simulink model "bipedal_robot_CTRL2"  (R2020b)
settings: Solver=ode23  StartTime=0.0  StopTime=Tsim  MaxStep=0.01  RelTol=1e-3  AbsTol=1e-3  EnableMultiTasking=on
values from neighbouring files (symbols this model uses):
  g = 9.80665    [bipedal.m]
  Tfil = Ts*10    (= 0.01)    [bipedal.m]
  total_mass = mlist(1) + ll_mass + rl_mass    [bipedal.m]
  Ts = 1/fs    (= 0.001)    [bipedal.m]
undefined symbols (not defined in the file or in its folder): Base, ctrl_cfg_rem, Fdist, LefAnklePitch, LefAnkleRoll, LefHipPitch, LefHipRoll, LefHipYaw, LefKnee, pg_traj, RigAnklePitch, RigAnkleRoll, RigHipPitch, RigHipRoll, RigHipYaw, RigKnee, sim_floor, Tdist, VAR_DIST, X, Y, Z
libraries: sm_lib x56, biped_lib x39, nesl_utility x18, simulink x3, Contact_Forces_Lib x2, robotmaniplib x1
(part 3 of 4)

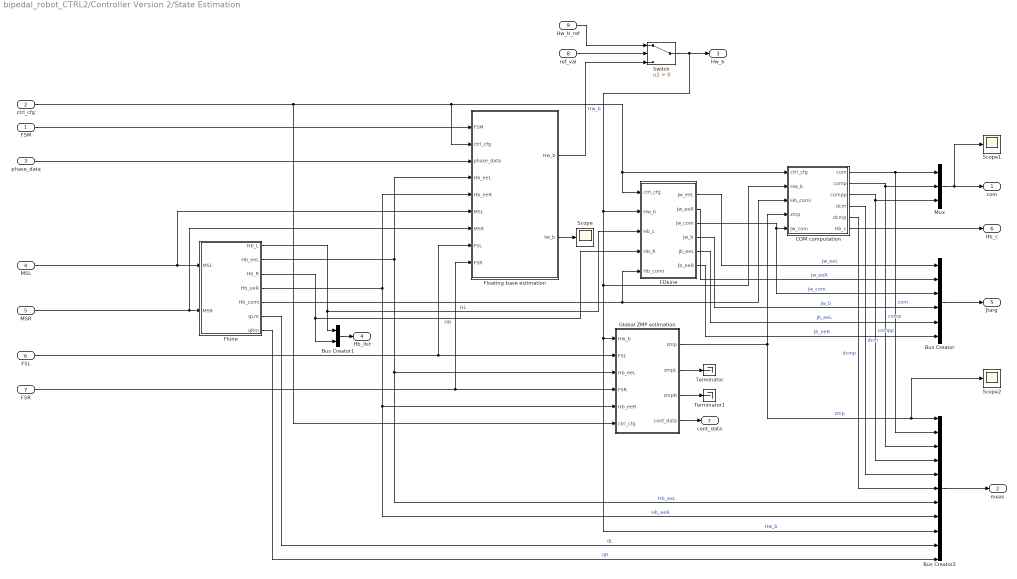
== system bipedal_robot_CTRL2/Controller Version 2/State Estimation ==
  FSM : Inport
  ctrl_cfg : Inport  Port=2
  phase_data : Inport  Port=3  OutDataTypeStr=Bus: ph_data_bus
  MSL : Inport  Port=4
  MSR : Inport  Port=5
  FSL : Inport  Port=6  OutDataTypeStr=Bus: fs_str_bus
  FSR : Inport  Port=7  OutDataTypeStr=Bus: fs_str_bus
  ref_val : Inport  Port=8
  Hw_b_ref : Inport  Port=9
  Bus Creator : BusCreator  Inputs=6  OutDataTypeStr=Bus: jac_bus
  Bus Creator1 : BusCreator  Inputs=2
  Bus Creator2 : BusCreator  Inputs=11  OutDataTypeStr=Bus: meas_bus
  COM computation : MATLAB Function  TreatAsAtomicUnit=on
  FDkine : MATLAB Function  TreatAsAtomicUnit=on
  Fkine : MATLAB Function  TreatAsAtomicUnit=on
  Floating base estimation : MATLAB Function  TreatAsAtomicUnit=on
  Global ZMP estimation : MATLAB Function  TreatAsAtomicUnit=on
  Mux : Mux  Inputs=3
  Scope : Scope
  Scope1 : Scope
  Scope2 : Scope
  Switch : Switch  Criteria=u2 > Threshold
  Terminator : Terminator
  Terminator1 : Terminator
  com : Outport
  meas : Outport  Port=2
  Hw_b : Outport  Port=3
  Hb_list : Outport  Port=4
  Jtarg : Outport  Port=5
  Hb_c : Outport  Port=6
  cont_data : Outport  Port=7
  wires:
  Bus Creator2/1 -> meas/1
  Fkine/7(qRm) -> Bus Creator2/11  "qR"
  Fkine/6(qLm) -> Bus Creator2/10  "qL"
  Fkine/4(Hb_eeR) -> Bus Creator2/8, Global ZMP estimation/5(Hb_eeR), Floating base estimation/5(Hb_eeR)  "Hb_eeR"
  Fkine/2(Hb_eeL) -> Bus Creator2/7, Global ZMP estimation/3(Hb_eeL), Floating base estimation/4(Hb_eeL)  "Hb_eeL"
  COM computation/5(dcmp) -> Bus Creator2/6  "dcmp"
  COM computation/4(dcm) -> Bus Creator2/5  "dcm"
  COM computation/3(compp) -> Bus Creator2/4, Mux/3  "compp"
  COM computation/2(comp) -> Bus Creator2/3, Mux/2  "comp"
  COM computation/1(com) -> Bus Creator2/2, Mux/1  "com"
  Bus Creator1/1 -> Hb_list/1
  Global ZMP estimation/3(zmpR) -> Terminator1/1
  Global ZMP estimation/2(zmpL) -> Terminator/1
  MSR/1 -> Fkine/2(MSR), Floating base estimation/7(MSR)
  MSL/1 -> Fkine/1(MSL), Floating base estimation/6(MSL)
  Global ZMP estimation/1(zmp) -> COM computation/4(zmp), Scope2/1, Bus Creator2/1  "zmp"
  ctrl_cfg/1 -> Global ZMP estimation/6(ctrl_cfg), Floating base estimation/2(ctrl_cfg), COM computation/1(ctrl_cfg), FDkine/1(ctrl_cfg)
  Bus Creator/1 -> Jtarg/1
  FDkine/4(Jw_b) -> Bus Creator/4  "Jw_b"
  FDkine/2(Jw_eeR) -> Bus Creator/2  "Jw_eeR"
  FDkine/1(Jw_eeL) -> Bus Creator/1  "Jw_eeL"
  FDkine/3(Jw_com) -> Bus Creator/3, COM computation/5(Jw_com)  "Jw_com"
  Fkine/5(Hb_comi) -> COM computation/3(Hb_comi), FDkine/5(Hb_comi)
  Switch/1 -> Hw_b/1, FDkine/2(Hw_b), Bus Creator2/9, Global ZMP estimation/1(Hw_b), COM computation/2(Hw_b)  "Hw_b"
  FSM/1 -> Floating base estimation/1(FSM)
  phase_data/1 -> Floating base estimation/3(phase_data)
  Fkine/3(Hb_R) -> FDkine/4(Hb_R), Bus Creator1/2  "HR"
  Fkine/1(Hb_L) -> FDkine/3(Hb_L), Bus Creator1/1  "HL"
  FSR/1 -> Floating base estimation/9(FSR), Global ZMP estimation/4(FSR)
  FSL/1 -> Floating base estimation/8(FSL), Global ZMP estimation/2(FSL)
  Floating base estimation/2(tw_b) -> Scope/1
  ref_val/1 -> Switch/2
  Hw_b_ref/1 -> Switch/1
  Floating base estimation/1(Hw_b) -> Switch/3  "Hw_b"
  FDkine/5(Jb_eeL) -> Bus Creator/5  "Jb_eeL"
  FDkine/6(Jb_eeR) -> Bus Creator/6  "Jb_eeR"
  COM computation/6(Hb_c) -> Hb_c/1
  Mux/1 -> Scope1/1, com/1
  Global ZMP estimation/4(cont_data) -> cont_data/1

== system bipedal_robot_CTRL2/Controller Version 2/Static spring force compensation (internal forces) ==
  ctrl_cfg : Inport
  qL : Inport  Port=2
  qR : Inport  Port=3
  HL_list : Inport  Port=4
  HR_list : Inport  Port=5
  Bungee cord compensation : MATLAB Function  TreatAsAtomicUnit=on
  Gas spring compensation : MATLAB Function  TreatAsAtomicUnit=on
  Sum2 : Sum  Inputs=|++
  Sum3 : Sum  Inputs=|++
  TL : Outport
  TR : Outport  Port=2
  wires:
  qR/1 -> Gas spring compensation/3(MSR)
  qL/1 -> Gas spring compensation/2(MSL)
  HR_list/1 -> Gas spring compensation/5(HR_list), Bungee cord compensation/3(HR_list)
  Gas spring compensation/2(TR) -> Sum3/1
  Gas spring compensation/1(TL) -> Sum2/1
  HL_list/1 -> Gas spring compensation/4(HL_list), Bungee cord compensation/2(HL_list)
  ctrl_cfg/1 -> Gas spring compensation/1(ctrl_cfg), Bungee cord compensation/1(ctrl_cfg)
  Bungee cord compensation/2(TR) -> Sum3/2
  Sum3/1 -> TR/1
  Sum2/1 -> TL/1
  Bungee cord compensation/1(TL) -> Sum2/2

== system bipedal_robot_CTRL2/Controller Version 2/Trajectory Generation ==
  note: 1) Add Subsystem or Model blocks as valid variant choices.
      | 2) You cannot connect blocks at this level. At simulation, connectivity is automatically
      | determined, based on the active variant and port name matching.
  FSM : Inport
  zmp_curr : Inport  Port=2
  com_m : Inport  Port=3
  (C++ impl) : Subsystem  VariantControl=VAR_TG == 2
  Preview Controller (simulink impl) : Subsystem  VariantControl=VAR_TG == 1
  tg_data : Outport  OutDataTypeStr=Bus: tg_out_bus

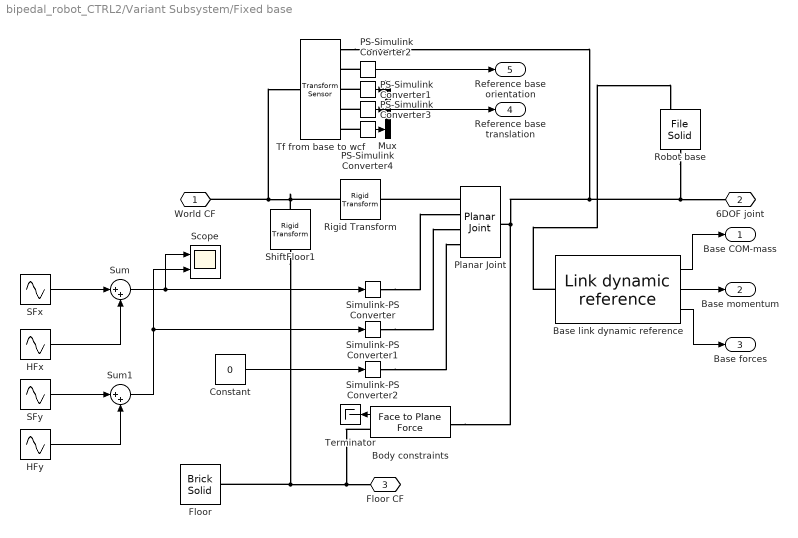
== system bipedal_robot_CTRL2/Variant Subsystem/Fixed base ==
  Base link dynamic reference : biped_lib/Link dynamic reference  M=Base.body.mass  I=Base.body.inertia
  Body constraints : Contact_Forces_Lib/3D/Composite Forces/Face to Plane Force  PlaB_x=sim_floor.dims(1)  PlaB_y=sim_floor.dims(2)  PlaB_z=sim_floor.dims(3)/2  FacF_x=Base.dims(1)  FacF_y=Base.dims(2)  FacF_z=Base.dims(3)/2  FacF_rSph=0.01  force_law_pla2pla=Linear  k_contact_pla2pla=Kcont  b_contact_pla2pla=Dcont  pen_full_damp_F_pla2pla=1e-4  pen_exponent_pla2pla=1  friction_law_pla2pla=Stick-Slip Continuous  mu_kinetic_pla2pla=0.5  mu_static_pla2pla=0.7  v_thr_pla2pla=0.001  vis_on_pla2pla=off  vis_opc_en_box2box=0  vis_len_plaLz=0.005  vis_clr=[0.9 0.2 0.2]  vis_opc=0.7
      settings: SourceProductName=Simscape Multibody Contact Forces Library
  Constant : Constant  Value=0
  Floor : sm_lib/Body Elements/Brick Solid  GraphicAmbientColor=[0.15 0.15 0.15 1.0]  BasedOnType=Density  BrickDimensions=sim_floor.dims  BrickDimensionUnits=m  CenterOfMass=[0 0 0]  CenterOfMassUnits=m  GraphicDiffuseColor=[0.8 0.8 0.8]  Density=1000  DensityUnits=kg/m^3  DoExposeReferenceFrame=on  GraphicEmissiveColor=[0.0 0.0 0.0 1.0]  ExportEntireGeometry=off  SerializedFrames=<Frames/>  MarkerShape=Sphere  MarkerSize=10  GraphicType=FromGeometry  InertiaType=CalculateFromGeometry  Mass=1  MassUnits=kg  MomentsOfInertia=[1 1 1]  MomentsOfInertiaUnits=kg*m^2  GraphicOpacity=1.0  ProductsOfInertia=[0 0 0]  ProductsOfInertiaUnits=kg*m^2  GraphicShininess=75  GraphicSpecularColor=[0.5 0.5 0.5 1.0]  GraphicVisPropType=SimpleVisualProperties
      settings: SourceProductName=Multibody
  HFx : Sin  Amplitude=0.001  Frequency=10  SampleTime=Ts
  HFy : Sin  Amplitude=0.001  Frequency=12  SampleTime=Ts
  Mux : Mux  Inputs=3
  PS-Simulink Converter{1..4} (4 alike) : nesl_utility/PS-Simulink Converter  PhysicalDomain=network_engine_domain  SubClassName=ps_output  LeftPortType=input  RightPortType=output  PseudoPeriodic=off  Frequencies=[]  Unit=1  AffineConversion=off
  Planar Joint : sm_lib/Joints/Planar Joint  JointMode=Normal  SenseConstraintForce=off  SenseConstraintForceX=off  SenseConstraintForceY=off  SenseConstraintForceZ=off  SenseConstraintTorque=off  SenseConstraintTorqueX=off  SenseConstraintTorqueY=off  SenseConstraintTorqueZ=off  SenseTotalForce=off  SenseTotalForceX=off  SenseTotalForceY=off  SenseTotalForceZ=off  SenseTotalTorque=off  SenseTotalTorqueX=off  SenseTotalTorqueY=off  SenseTotalTorqueZ=off  CompositeWrenchDir=FollowerOnBase  CompositeWrenchFrame=BaseFrame  PxEquilibriumPosition=0  PxEquilibriumPositionUnits=m  PxSpringStiffness=1000  PxSpringStiffnessUnits=N/m  PxDampingCoefficient=100  PxDampingCoefficientUnits=N/(m/s)  PxTorqueActuationMode=ComputedTorque  PxMotionActuationMode=InputMotion  PxSensePosition=off  PxSenseVelocity=off  PxSenseAcceleration=off  PxSenseTorqueForce=off  PxSenseLowerLimitTorqueForce=off  PxSenseUpperLimitTorqueForce=off  PxLowerLimitSpecify=off  PxLowerLimitBound=-1  PxLowerLimitBoundUnits=m  PxLowerLimitStiffness=1e6  PxLowerLimitStiffnessUnits=N/m  PxLowerLimitDamping=1e3  PxLowerLimitDampingUnits=N/(m/s)  PxLowerLimitTransitionRegionWidth=1e-4  PxLowerLimitTransitionRegionWidthUnits=m  PxUpperLimitSpecify=off  PxUpperLimitBound=1  PxUpperLimitBoundUnits=m  PxUpperLimitStiffness=1e6  PxUpperLimitStiffnessUnits=N/m  PxUpperLimitDamping=1e3  PxUpperLimitDampingUnits=N/(m/s)  PxUpperLimitTransitionRegionWidth=1e-4  PxUpperLimitTransitionRegionWidthUnits=m  PxPositionTargetSpecify=off  PxPositionTargetPriority=High  PxPositionTargetValue=0  PxPositionTargetValueUnits=m  PxVelocityTargetSpecify=off  PxVelocityTargetPriority=High  PxVelocityTargetValue=0  PxVelocityTargetValueUnits=m/s  PyEquilibriumPosition=0  PyEquilibriumPositionUnits=m  PySpringStiffness=1000  PySpringStiffnessUnits=N/m  PyDampingCoefficient=100  PyDampingCoefficientUnits=N/(m/s)  PyTorqueActuationMode=ComputedTorque  PyMotionActuationMode=InputMotion  PySensePosition=off  PySenseVelocity=off  PySenseAcceleration=off  PySenseTorqueForce=off  PySenseLowerLimitTorqueForce=off  PySenseUpperLimitTorqueForce=off  PyLowerLimitSpecify=off  PyLowerLimitBound=-1  PyLowerLimitBoundUnits=m  PyLowerLimitStiffness=1e6  PyLowerLimitStiffnessUnits=N/m  PyLowerLimitDamping=1e3  PyLowerLimitDampingUnits=N/(m/s)  PyLowerLimitTransitionRegionWidth=1e-4  PyLowerLimitTransitionRegionWidthUnits=m  PyUpperLimitSpecify=off  PyUpperLimitBound=1  PyUpperLimitBoundUnits=m  PyUpperLimitStiffness=1e6  PyUpperLimitStiffnessUnits=N/m  PyUpperLimitDamping=1e3  PyUpperLimitDampingUnits=N/(m/s)  PyUpperLimitTransitionRegionWidth=1e-4  PyUpperLimitTransitionRegionWidthUnits=m  PyPositionTargetSpecify=off  PyPositionTargetPriority=High  PyPositionTargetValue=0  PyPositionTargetValueUnits=m  PyVelocityTargetSpecify=off  PyVelocityTargetPriority=High  PyVelocityTargetValue=0  PyVelocityTargetValueUnits=m/s  RzEquilibriumPosition=0  RzEquilibriumPositionUnits=deg  RzSpringStiffness=1000  RzSpringStiffnessUnits=N*m/deg  RzDampingCoefficient=100  RzDampingCoefficientUnits=N*m/(deg/s)  RzTorqueActuationMode=ComputedTorque  RzMotionActuationMode=InputMotion  RzSensePosition=off  RzSenseVelocity=off  RzSenseAcceleration=off  RzSenseTorqueForce=off  RzSenseLowerLimitTorqueForce=off  RzSenseUpperLimitTorqueForce=off  RzLowerLimitSpecify=off  RzLowerLimitBound=-90  RzLowerLimitBoundUnits=deg  RzLowerLimitStiffness=1e4  RzLowerLimitStiffnessUnits=N*m/deg  RzLowerLimitDamping=10  RzLowerLimitDampingUnits=N*m/(deg/s)  RzLowerLimitTransitionRegionWidth=0.1  RzLowerLimitTransitionRegionWidthUnits=deg  RzUpperLimitSpecify=off  RzUpperLimitBound=90  RzUpperLimitBoundUnits=deg  RzUpperLimitStiffness=1e4  RzUpperLimitStiffnessUnits=N*m/deg  RzUpperLimitDamping=10  RzUpperLimitDampingUnits=N*m/(deg/s)  RzUpperLimitTransitionRegionWidth=0.1  RzUpperLimitTransitionRegionWidthUnits=deg  RzPositionTargetSpecify=off  RzPositionTargetPriority=High  RzPositionTargetValue=0  RzPositionTargetValueUnits=deg  RzVelocityTargetSpecify=off  RzVelocityTargetPriority=High  RzVelocityTargetValue=0  RzVelocityTargetValueUnits=deg/s
  Rigid Transform : sm_lib/Frames and Transforms/Rigid Transform  TranslationMethod=Cartesian  TranslationStandardOffset=Base.Xinit  TranslationLengthUnit=m  TranslationStandardAxis=+Z  TranslationCartesianOffset=Base.Xinit  TranslationROffset=0  TranslationROffsetUnits=m  TranslationZOffset=0  TranslationZOffsetUnits=m  TranslationThetaOffset=0  TranslationThetaOffsetUnits=deg  RotationMethod=None  RotationAngleUnits=deg  RotationStandardAxis=+Z  RotationAngle=0.0  RotationArbitraryAxis=[0 0 1]  FollAlignAxisA=+X  BaseAlignAxisA=+Y  FollAlignAxisB=+Y  BaseAlignAxisB=+Z  RotationSequenceAxes=FollowerAxes  RotationSequence=XYX  RotationSequenceAngles=[0 0 0]  RotationSequenceAnglesUnits=deg  RotationMatrix=[1 0 0; 0 1 0; 0 0 1]
  Robot base : sm_lib/Body Elements/File Solid  ExtGeomFileName=Base.stl  UnitType=Custom  ExtGeomFileUnits=mm  StepReaderType=HEX  ExportConvexHullGeometry=on  InertiaType=Custom  Mass=Base.body.mass  MassUnits=kg  CenterOfMass=Base.body.com  CenterOfMassUnits=m  MomentsOfInertia=Base.body.inertia(1:3)  MomentsOfInertiaUnits=kg*m^2  ProductsOfInertia=Base.body.inertia(4:6)  ProductsOfInertiaUnits=kg*m^2  BasedOnType=Mass  Density=1000  DensityUnits=kg/m^3  DoExposeReferenceFrame=on  SerializedFrames=<Frames><Frame><Id>Frame1</Id><Value><Name>COM</Name><Origin><Source>CenterOfMassFrame</Source><FeatureName></FeatureName></Origin><PrimaryAxis><DefinedDirection>+Z</DefinedDirection><Source>ReferenceFrame</Source><SourceDirection>+Z</SourceDirection><FeatureName></FeatureName></PrimaryAxis><SecondaryAxis><DefinedDirection>+X</DefinedDirection><Source>ReferenceFrame</Source><SourceDirection>+X</SourceDirection><FeatureName></FeatureName></SecondaryAxis></Value></Frame></Frames>  GraphicType=FromGeometry  MarkerShape=Sphere  MarkerSize=10  GraphicVisPropType=SimpleVisualProperties  GraphicDiffuseColor=[0.5 0.5 0.5]  GraphicSpecularColor=[0.5 0.5 0.5 1.0]  GraphicAmbientColor=[0.15 0.15 0.15 1.0]  GraphicEmissiveColor=[0.0 0.0 0.0 1.0]  GraphicShininess=75  GraphicOpacity=1.0
  SFx : Sin  Amplitude=0.2  Frequency=0.5  SampleTime=Ts
  SFy : Sin  Amplitude=0.1  SampleTime=Ts
  Scope : Scope  NumInputPorts=2
  ShiftFloor1 : sm_lib/Frames and Transforms/Rigid Transform  TranslationMethod=StandardAxis  TranslationStandardOffset=-sim_floor.dims(3)/2*5  TranslationLengthUnit=m  TranslationStandardAxis=+Z  TranslationCartesianOffset=[0 0 0]  TranslationROffset=0  TranslationROffsetUnits=m  TranslationZOffset=0  TranslationZOffsetUnits=m  TranslationThetaOffset=0  TranslationThetaOffsetUnits=deg  RotationMethod=None  RotationAngleUnits=deg  RotationStandardAxis=+Z  RotationAngle=0.0  RotationArbitraryAxis=[0 0 1]  FollAlignAxisA=+X  BaseAlignAxisA=+Y  FollAlignAxisB=+Y  BaseAlignAxisB=+Z  RotationSequenceAxes=FollowerAxes  RotationSequence=XYX  RotationSequenceAngles=[0 0 0]  RotationSequenceAnglesUnits=deg  RotationMatrix=[1 0 0; 0 1 0; 0 0 1]
  Simulink-PS Converter : nesl_utility/Simulink-PS Converter  PhysicalDomain=network_engine_domain  SubClassName=ps_input  LeftPortType=input  RightPortType=output  PseudoPeriodic=off  Frequencies=[]  NoiseDistribution=none  NoiseParameters=[]  Unit=1  AffineConversion=off  FilteringAndDerivatives=filter  SimscapeFilterOrder=2  InputFilterTimeConstant=0.001  UdotUserProvided=0
      settings: SourceProductName=Utilities
  Simulink-PS Converter1 : nesl_utility/Simulink-PS Converter  PhysicalDomain=network_engine_domain  SubClassName=ps_input  LeftPortType=input  RightPortType=output  PseudoPeriodic=off  Frequencies=[]  NoiseDistribution=none  NoiseParameters=[]  Unit=1  AffineConversion=off  FilteringAndDerivatives=filter  SimscapeFilterOrder=2  InputFilterTimeConstant=0.001  UdotUserProvided=0
      settings: SourceProductName=Utilities
  Simulink-PS Converter2 : nesl_utility/Simulink-PS Converter  PhysicalDomain=network_engine_domain  SubClassName=ps_input  LeftPortType=input  RightPortType=output  PseudoPeriodic=off  Frequencies=[]  NoiseDistribution=none  NoiseParameters=[]  Unit=1  AffineConversion=off  FilteringAndDerivatives=filter  SimscapeFilterOrder=2  InputFilterTimeConstant=0.001  UdotUserProvided=0
      settings: SourceProductName=Utilities
  Sum : Sum  Inputs=|++
  Sum1 : Sum  Inputs=|++
  Terminator : Terminator
  Tf from base to wcf : sm_lib/Frames and Transforms/Transform Sensor  MeasurementFrame=World  SenseAngle=off  SenseAxis=off  SenseAngle1=off  SenseAngle2=off  SenseAngle3=off  SenseQ=off  SenseR=on  SenseOmegaX=off  SenseOmegaY=off  SenseOmegaZ=off  SenseOmega1=off  SenseOmega2=off  SenseOmega3=off  SenseQDot=off  SenseRDot=off  SenseAlphaX=off  SenseAlphaY=off  SenseAlphaZ=off  SenseAlpha1=off  SenseAlpha2=off  SenseAlpha3=off  SenseQDDot=off  SenseRDDot=off  SenseX=on  SenseY=on  SenseZ=on  SenseRad=off  SenseAzim=off  SenseDist=off  SenseInc=off  SenseXDot=off  SenseYDot=off  SenseZDot=off  SenseRadDot=off  SenseAzimDot=off  SenseDistDot=off  SenseIncDot=off  SenseXDDot=off  SenseYDDot=off  SenseZDDot=off  SenseRadDDot=off  SenseAzimDDot=off  SenseDistDDot=off  SenseIncDDot=off
  World CF : PMIOPort  Side=Left
  6DOF joint : PMIOPort  Port=2  Side=Right
  Floor CF : PMIOPort  Port=3  Side=Right
  Base COM-mass : Outport
  Base momentum : Outport  Port=2
  Base forces : Outport  Port=3
  Reference base translation : Outport  Port=4
  Reference base orientation : Outport  Port=5
  wires:
  Mux/1 -> Reference base translation/1
  PS-Simulink Converter4/1 -> Mux/3
  PS-Simulink Converter1/1 -> Mux/1
  PS-Simulink Converter3/1 -> Mux/2
  PS-Simulink Converter2/1 -> Reference base orientation/1
  Base link dynamic reference/3 -> Base forces/1
  Base link dynamic reference/2 -> Base momentum/1
  Base link dynamic reference/1 -> Base COM-mass/1
  Body constraints/1 -> Terminator/1
  Sum/1 -> Simulink-PS Converter/1, Scope/1
  Sum1/1 -> Simulink-PS Converter1/1, Scope/2
  Constant/1 -> Simulink-PS Converter2/1
  SFy/1 -> Sum1/1
  HFy/1 -> Sum1/2
  HFx/1 -> Sum/2
  SFx/1 -> Sum/1
  connections:
  Base link dynamic reference/LConn1 -- Robot base/LConn1
  PS-Simulink Converter4/LConn1 -- Tf from base to wcf/RConn5
  PS-Simulink Converter3/LConn1 -- Tf from base to wcf/RConn4
  PS-Simulink Converter1/LConn1 -- Tf from base to wcf/RConn3
  PS-Simulink Converter2/LConn1 -- Tf from base to wcf/RConn2
  Body constraints/RConn1 -- Floor CF/RConn1 -- Floor/RConn1 -- ShiftFloor1/RConn1
  Robot base/RConn1 -- 6DOF joint/RConn1 -- Tf from base to wcf/RConn1 -- Body constraints/LConn1 -- Planar Joint/RConn1
  ShiftFloor1/LConn1 -- World CF/RConn1 -- Tf from base to wcf/LConn1 -- Rigid Transform/LConn1
  Planar Joint/LConn1 -- Rigid Transform/RConn1
  Simulink-PS Converter/RConn1 -- Planar Joint/LConn2
  Simulink-PS Converter1/RConn1 -- Planar Joint/LConn3
  Simulink-PS Converter2/RConn1 -- Planar Joint/LConn4

== system bipedal_robot_CTRL2/Variant Subsystem/Floating base ==
  6-DOF Joint : sm_lib/Joints/6-DOF Joint  JointMode=Normal  SenseConstraintForce=off  SenseConstraintForceX=off  SenseConstraintForceY=off  SenseConstraintForceZ=off  SenseConstraintTorque=off  SenseConstraintTorqueX=off  SenseConstraintTorqueY=off  SenseConstraintTorqueZ=off  SenseTotalForce=off  SenseTotalForceX=off  SenseTotalForceY=off  SenseTotalForceZ=off  SenseTotalTorque=off  SenseTotalTorqueX=off  SenseTotalTorqueY=off  SenseTotalTorqueZ=off  CompositeWrenchDir=FollowerOnBase  CompositeWrenchFrame=BaseFrame  PxEquilibriumPosition=0  PxEquilibriumPositionUnits=m  PxSpringStiffness=0  PxSpringStiffnessUnits=N/m  PxDampingCoefficient=0  PxDampingCoefficientUnits=N/(m/s)  PxTorqueActuationMode=NoTorque  PxMotionActuationMode=ComputedMotion  PxSensePosition=off  PxSenseVelocity=off  PxSenseAcceleration=off  PxSenseTorqueForce=off  PxSenseLowerLimitTorqueForce=off  PxSenseUpperLimitTorqueForce=off  PxLowerLimitSpecify=off  PxLowerLimitBound=-1  PxLowerLimitBoundUnits=m  PxLowerLimitStiffness=1e6  PxLowerLimitStiffnessUnits=N/m  PxLowerLimitDamping=1e3  PxLowerLimitDampingUnits=N/(m/s)  PxLowerLimitTransitionRegionWidth=1e-4  PxLowerLimitTransitionRegionWidthUnits=m  PxUpperLimitSpecify=off  PxUpperLimitBound=1  PxUpperLimitBoundUnits=m  PxUpperLimitStiffness=1e6  PxUpperLimitStiffnessUnits=N/m  PxUpperLimitDamping=1e3  PxUpperLimitDampingUnits=N/(m/s)  PxUpperLimitTransitionRegionWidth=1e-4  PxUpperLimitTransitionRegionWidthUnits=m  PxPositionTargetSpecify=on  PxPositionTargetPriority=High  PxPositionTargetValue=Base.Xinit(1)  PxPositionTargetValueUnits=m  PxVelocityTargetSpecify=off  PxVelocityTargetPriority=High  PxVelocityTargetValue=0  PxVelocityTargetValueUnits=m/s  PyEquilibriumPosition=0  PyEquilibriumPositionUnits=m  PySpringStiffness=0  PySpringStiffnessUnits=N/m  PyDampingCoefficient=0  PyDampingCoefficientUnits=N/(m/s)  PyTorqueActuationMode=NoTorque  PyMotionActuationMode=ComputedMotion  PySensePosition=off  PySenseVelocity=off  PySenseAcceleration=off  PySenseTorqueForce=off  PySenseLowerLimitTorqueForce=off  PySenseUpperLimitTorqueForce=off  PyLowerLimitSpecify=off  PyLowerLimitBound=-1  PyLowerLimitBoundUnits=m  PyLowerLimitStiffness=1e6  PyLowerLimitStiffnessUnits=N/m  PyLowerLimitDamping=1e3  PyLowerLimitDampingUnits=N/(m/s)  PyLowerLimitTransitionRegionWidth=1e-4  PyLowerLimitTransitionRegionWidthUnits=m  PyUpperLimitSpecify=off  PyUpperLimitBound=1  PyUpperLimitBoundUnits=m  PyUpperLimitStiffness=1e6  PyUpperLimitStiffnessUnits=N/m  PyUpperLimitDamping=1e3  PyUpperLimitDampingUnits=N/(m/s)  PyUpperLimitTransitionRegionWidth=1e-4  PyUpperLimitTransitionRegionWidthUnits=m  PyPositionTargetSpecify=on  PyPositionTargetPriority=High  PyPositionTargetValue=Base.Xinit(2)  PyPositionTargetValueUnits=m  PyVelocityTargetSpecify=off  PyVelocityTargetPriority=High  PyVelocityTargetValue=0  PyVelocityTargetValueUnits=m/s  PzEquilibriumPosition=0  PzEquilibriumPositionUnits=m  PzSpringStiffness=0  PzSpringStiffnessUnits=N/m  PzDampingCoefficient=0  PzDampingCoefficientUnits=N/(m/s)  PzTorqueActuationMode=NoTorque  PzMotionActuationMode=ComputedMotion  PzSensePosition=off  PzSenseVelocity=off  PzSenseAcceleration=off  PzSenseTorqueForce=off  PzSenseLowerLimitTorqueForce=off  PzSenseUpperLimitTorqueForce=off  PzLowerLimitSpecify=off  PzLowerLimitBound=0  PzLowerLimitBoundUnits=m  PzLowerLimitStiffness=1e6  PzLowerLimitStiffnessUnits=N/m  PzLowerLimitDamping=1e3  PzLowerLimitDampingUnits=N/(m/s)  PzLowerLimitTransitionRegionWidth=1e-4  PzLowerLimitTransitionRegionWidthUnits=m  PzUpperLimitSpecify=off  PzUpperLimitBound=1  PzUpperLimitBoundUnits=m  PzUpperLimitStiffness=1e6  PzUpperLimitStiffnessUnits=N/m  PzUpperLimitDamping=1e3  PzUpperLimitDampingUnits=N/(m/s)  PzUpperLimitTransitionRegionWidth=1e-4  PzUpperLimitTransitionRegionWidthUnits=m  PzPositionTargetSpecify=on  PzPositionTargetPriority=High  PzPositionTargetValue=Base.Xinit(3)  PzPositionTargetValueUnits=m  PzVelocityTargetSpecify=off  PzVelocityTargetPriority=High  PzVelocityTargetValue=0  PzVelocityTargetValueUnits=m/s  SphDefPosRotationMethod=None  SphDefPosRotationAngleUnits=deg  SphDefPosRotationStandardAxis=+Z  SphDefPosRotationAngle=0.0  SphDefPosRotationArbitraryAxis=[0 0 1]  SphDefPosFollAlignAxisA=+X  SphDefPosBaseAlignAxisA=+Y  SphDefPosFollAlignAxisB=+Y  SphDefPosBaseAlignAxisB=+Z  SphDefPosRotationSequenceAxes=FollowerAxes  SphDefPosRotationSequence=XYX  SphDefPosRotationSequenceAngles=[0 0 0]  SphDefPosRotationSequenceAnglesUnits=deg  SphDefPosRotationMatrix=[1 0 0; 0 1 0; 0 0 1]  SphEqPosRotationMethod=None  SphEqPosRotationAngleUnits=deg  SphEqPosRotationStandardAxis=+Z  SphEqPosRotationAngle=0.0  SphEqPosRotationArbitraryAxis=[0 0 1]  SphEqPosFollAlignAxisA=+X  SphEqPosBaseAlignAxisA=+Y  SphEqPosFollAlignAxisB=+Y  SphEqPosBaseAlignAxisB=+Z  SphEqPosRotationSequenceAxes=FollowerAxes  SphEqPosRotationSequence=XYX  SphEqPosRotationSequenceAngles=[0 0 0]  SphEqPosRotationSequenceAnglesUnits=deg  SphEqPosRotationMatrix=[1 0 0; 0 1 0; 0 0 1]  SphSpringStiffness=0  SphSpringStiffnessUnits=N*m/deg  SphDampingCoefficient=0  SphDampingCoefficientUnits=N*m/(deg/s)  SphActuateTorqueX=off  SphActuateTorqueY=off  SphActuateTorqueZ=off  SphActuateTorque=off  SphTorqueActuationMode=NoTorque  SphMotionActuationMode=ComputedMotion  SphActuationFrame=BaseFrame  SphSensePosition=off  SphSenseVelocityX=off  SphSenseVelocityY=off  SphSenseVelocityZ=off  SphSenseVelocity=off  SphSenseAccelerationX=off  SphSenseAccelerationY=off  SphSenseAccelerationZ=off  SphSenseAcceleration=off  SphSenseTorqueX=off  SphSenseTorqueY=off  SphSenseTorqueZ=off  SphSenseTorqueForce=off  SphSenseLowerLimitTorqueMag=off  SphSenseUpperLimitTorqueMag=off  SphSensingFrame=BaseFrame  SphLowerLimitSpecify=off  SphLowerLimitBound=15  SphLowerLimitBoundUnits=deg  SphLowerLimitStiffness=1e4  SphLowerLimitStiffnessUnits=N*m/deg  SphLowerLimitDamping=10  SphLowerLimitDampingUnits=N*m/(deg/s)  SphLowerLimitTransitionRegionWidth=0.1  SphLowerLimitTransitionRegionWidthUnits=deg  SphUpperLimitSpecify=off  SphUpperLimitBound=45  SphUpperLimitBoundUnits=deg  SphUpperLimitStiffness=1e4  SphUpperLimitStiffnessUnits=N*m/deg  SphUpperLimitDamping=10  SphUpperLimitDampingUnits=N*m/(deg/s)  SphUpperLimitTransitionRegionWidth=0.1  SphUpperLimitTransitionRegionWidthUnits=deg  SphPositionTargetRotationMethod=StandardAxis  SphPositionTargetRotationAngleUnits=rad  SphPositionTargetRotationStandardAxis=+Y  SphPositionTargetRotationAngle=0  SphPositionTargetRotationArbitraryAxis=[0 0 1]  SphPositionTargetFollAlignAxisA=+X  SphPositionTargetBaseAlignAxisA=+Y  SphPositionTargetFollAlignAxisB=+Y  SphPositionTargetBaseAlignAxisB=+Z  SphPositionTargetRotationSequenceAxes=FollowerAxes  SphPositionTargetRotationSequence=XYX  SphPositionTargetRotationSequenceAngles=[0 0 0]  SphPositionTargetRotationSequenceAnglesUnits=deg  SphPositionTargetRotationMatrix=[1 0 0; 0 1 0; 0 0 1]  SphPositionTargetSpecify=on  SphPositionTargetPriority=High  SphVelocityTargetValue=[0 0 0]  SphVelocityTargetValueUnits=deg/s  SphVelocityTargetSpecify=off  SphVelocityTargetPriority=High  SphVelocityTargetInFollowerFrame=on
  Base link dynamic reference : biped_lib/Link dynamic reference  M=Base.body.mass  I=Base.body.inertia
  Body constraints : Contact_Forces_Lib/3D/Composite Forces/Face to Plane Force  PlaB_x=sim_floor.dims(1)  PlaB_y=sim_floor.dims(2)  PlaB_z=sim_floor.dims(3)/2  FacF_x=Base.dims(1)  FacF_y=Base.dims(2)  FacF_z=Base.dims(3)/2  FacF_rSph=0.01  force_law_pla2pla=Linear  k_contact_pla2pla=Kcont  b_contact_pla2pla=Dcont  pen_full_damp_F_pla2pla=1e-4  pen_exponent_pla2pla=1  friction_law_pla2pla=Stick-Slip Continuous  mu_kinetic_pla2pla=0.5  mu_static_pla2pla=0.7  v_thr_pla2pla=0.001  vis_on_pla2pla=off  vis_opc_en_box2box=0  vis_len_plaLz=0.005  vis_clr=[0.9 0.2 0.2]  vis_opc=0.7
      settings: SourceProductName=Simscape Multibody Contact Forces Library
  Disturbance generator : Subsystem
  Floor : sm_lib/Body Elements/Brick Solid  GraphicAmbientColor=[0.15 0.15 0.15 1.0]  BasedOnType=Density  BrickDimensions=sim_floor.dims  BrickDimensionUnits=m  CenterOfMass=[0 0 0]  CenterOfMassUnits=m  GraphicDiffuseColor=[0.8 0.8 0.8]  Density=1000  DensityUnits=kg/m^3  DoExposeReferenceFrame=on  GraphicEmissiveColor=[0.0 0.0 0.0 1.0]  ExportEntireGeometry=off  SerializedFrames=<Frames/>  MarkerShape=Sphere  MarkerSize=10  GraphicType=FromGeometry  InertiaType=CalculateFromGeometry  Mass=1  MassUnits=kg  MomentsOfInertia=[1 1 1]  MomentsOfInertiaUnits=kg*m^2  GraphicOpacity=1.0  ProductsOfInertia=[0 0 0]  ProductsOfInertiaUnits=kg*m^2  GraphicShininess=75  GraphicSpecularColor=[0.5 0.5 0.5 1.0]  GraphicVisPropType=SimpleVisualProperties
      settings: SourceProductName=Multibody
  Mux : Mux  Inputs=3
  PS-Simulink Converter{1..4} (4 alike) : nesl_utility/PS-Simulink Converter  PhysicalDomain=network_engine_domain  SubClassName=ps_output  LeftPortType=input  RightPortType=output  PseudoPeriodic=off  Frequencies=[]  Unit=1  AffineConversion=off
  Rigid Transform : sm_lib/Frames and Transforms/Rigid Transform  TranslationMethod=StandardAxis  TranslationStandardOffset=0  TranslationLengthUnit=m  TranslationStandardAxis=+Z  TranslationCartesianOffset=[0 0 0]  TranslationROffset=0  TranslationROffsetUnits=m  TranslationZOffset=0  TranslationZOffsetUnits=m  TranslationThetaOffset=0  TranslationThetaOffsetUnits=deg  RotationMethod=None  RotationAngleUnits=deg  RotationStandardAxis=+Z  RotationAngle=0.0  RotationArbitraryAxis=[0 0 1]  FollAlignAxisA=+X  BaseAlignAxisA=+Y  FollAlignAxisB=+Y  BaseAlignAxisB=+Z  RotationSequenceAxes=FollowerAxes  RotationSequence=XYX  RotationSequenceAngles=[0 0 0]  RotationSequenceAnglesUnits=deg  RotationMatrix=[1 0 0; 0 1 0; 0 0 1]
  Robot base : sm_lib/Body Elements/File Solid  ExtGeomFileName=Base.stl  UnitType=Custom  ExtGeomFileUnits=mm  StepReaderType=HEX  ExportConvexHullGeometry=on  InertiaType=Custom  Mass=Base.body.mass  MassUnits=kg  CenterOfMass=Base.body.com  CenterOfMassUnits=m  MomentsOfInertia=Base.body.inertia(1:3)  MomentsOfInertiaUnits=kg*m^2  ProductsOfInertia=Base.body.inertia(4:6)  ProductsOfInertiaUnits=kg*m^2  BasedOnType=Mass  Density=1000  DensityUnits=kg/m^3  DoExposeReferenceFrame=on  SerializedFrames=<Frames><Frame><Id>Frame1</Id><Value><Name>COM</Name><Origin><Source>CenterOfMassFrame</Source><FeatureName></FeatureName></Origin><PrimaryAxis><DefinedDirection>+Z</DefinedDirection><Source>ReferenceFrame</Source><SourceDirection>+Z</SourceDirection><FeatureName></FeatureName></PrimaryAxis><SecondaryAxis><DefinedDirection>+X</DefinedDirection><Source>ReferenceFrame</Source><SourceDirection>+X</SourceDirection><FeatureName></FeatureName></SecondaryAxis></Value></Frame></Frames>  GraphicType=FromGeometry  MarkerShape=Sphere  MarkerSize=10  GraphicVisPropType=SimpleVisualProperties  GraphicDiffuseColor=[0.5 0.5 0.5]  GraphicSpecularColor=[0.5 0.5 0.5 1.0]  GraphicAmbientColor=[0.15 0.15 0.15 1.0]  GraphicEmissiveColor=[0.0 0.0 0.0 1.0]  GraphicShininess=75  GraphicOpacity=1.0
  ShiftFloor1 : sm_lib/Frames and Transforms/Rigid Transform  TranslationMethod=StandardAxis  TranslationStandardOffset=-sim_floor.dims(3)/2  TranslationLengthUnit=m  TranslationStandardAxis=+Z  TranslationCartesianOffset=[0 0 0]  TranslationROffset=0  TranslationROffsetUnits=m  TranslationZOffset=0  TranslationZOffsetUnits=m  TranslationThetaOffset=0  TranslationThetaOffsetUnits=deg  RotationMethod=None  RotationAngleUnits=deg  RotationStandardAxis=+Z  RotationAngle=0.0  RotationArbitraryAxis=[0 0 1]  FollAlignAxisA=+X  BaseAlignAxisA=+Y  FollAlignAxisB=+Y  BaseAlignAxisB=+Z  RotationSequenceAxes=FollowerAxes  RotationSequence=XYX  RotationSequenceAngles=[0 0 0]  RotationSequenceAnglesUnits=deg  RotationMatrix=[1 0 0; 0 1 0; 0 0 1]
  Terminator : Terminator
  Tf from base to wcf : sm_lib/Frames and Transforms/Transform Sensor  MeasurementFrame=World  SenseAngle=off  SenseAxis=off  SenseAngle1=off  SenseAngle2=off  SenseAngle3=off  SenseQ=off  SenseR=on  SenseOmegaX=off  SenseOmegaY=off  SenseOmegaZ=off  SenseOmega1=off  SenseOmega2=off  SenseOmega3=off  SenseQDot=off  SenseRDot=off  SenseAlphaX=off  SenseAlphaY=off  SenseAlphaZ=off  SenseAlpha1=off  SenseAlpha2=off  SenseAlpha3=off  SenseQDDot=off  SenseRDDot=off  SenseX=on  SenseY=on  SenseZ=on  SenseRad=off  SenseAzim=off  SenseDist=off  SenseInc=off  SenseXDot=off  SenseYDot=off  SenseZDot=off  SenseRadDot=off  SenseAzimDot=off  SenseDistDot=off  SenseIncDot=off  SenseXDDot=off  SenseYDDot=off  SenseZDDot=off  SenseRadDDot=off  SenseAzimDDot=off  SenseDistDDot=off  SenseIncDDot=off
  World CF : PMIOPort  Side=Left
  6DOF joint : PMIOPort  Port=2  Side=Right
  Floor CF : PMIOPort  Port=3  Side=Right
  Base COM-mass : Outport
  Base momentum : Outport  Port=2
  Base forces : Outport  Port=3
  Reference base translation : Outport  Port=4
  Reference base orientation : Outport  Port=5
  wires:
  Body constraints/1 -> Terminator/1
  Base link dynamic reference/1 -> Base COM-mass/1
  Base link dynamic reference/2 -> Base momentum/1
  Base link dynamic reference/3 -> Base forces/1
  PS-Simulink Converter2/1 -> Reference base orientation/1
  PS-Simulink Converter3/1 -> Mux/2
  PS-Simulink Converter1/1 -> Mux/1
  PS-Simulink Converter4/1 -> Mux/3
  Mux/1 -> Reference base translation/1
  connections:
  Rigid Transform/LConn1 -- Tf from base to wcf/LConn1 -- World CF/RConn1 -- ShiftFloor1/LConn1
  Rigid Transform/RConn1 -- 6-DOF Joint/LConn1
  6-DOF Joint/RConn1 -- Body constraints/LConn1 -- Disturbance generator/RConn1 -- Tf from base to wcf/RConn1 -- Robot base/RConn1 -- 6DOF joint/RConn1
  ShiftFloor1/RConn1 -- Floor/RConn1 -- Floor CF/RConn1 -- Body constraints/RConn1
  PS-Simulink Converter2/LConn1 -- Tf from base to wcf/RConn2
  PS-Simulink Converter1/LConn1 -- Tf from base to wcf/RConn3
  PS-Simulink Converter3/LConn1 -- Tf from base to wcf/RConn4
  PS-Simulink Converter4/LConn1 -- Tf from base to wcf/RConn5
  Base link dynamic reference/LConn1 -- Robot base/LConn1

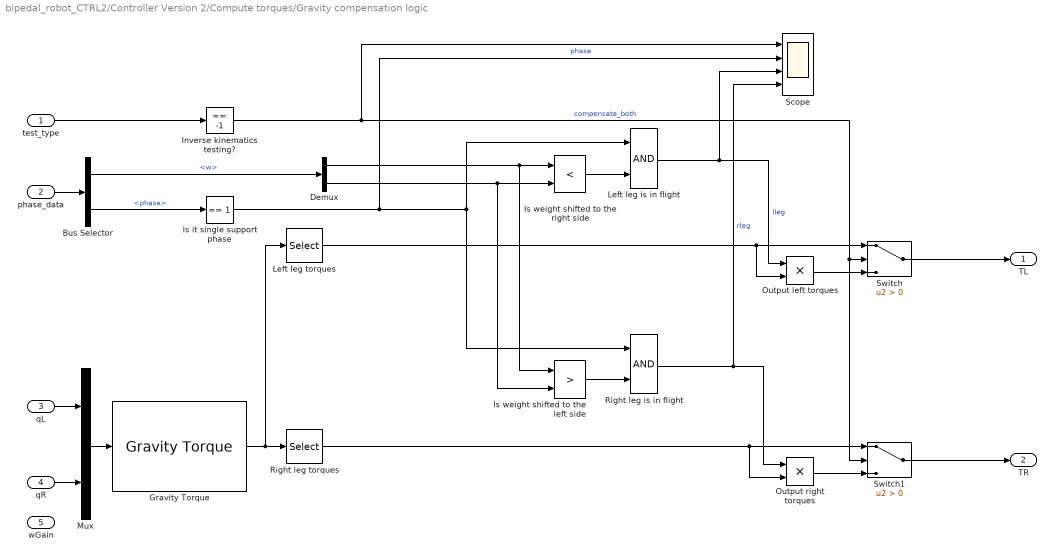
== system bipedal_robot_CTRL2/Controller Version 2/Compute torques/Gravity compensation logic ==
  test_type : Inport
  phase_data : Inport  Port=2
  qL : Inport  Port=3
  qR : Inport  Port=4
  wGain : Inport  Port=5
  Bus Selector : BusSelector  OutputSignals=w,phase
  Demux : Demux  Outputs=2
  Gravity Torque : robotmaniplib/Gravity Torque  RigidBodyTree=roby  SimulateUsing=Code generation
  Inverse kinematics testing? : simulink/Logic and Bit Operations/Compare To Constant  relop===  const=-1  OutDataTypeStr=boolean
  Is it single support phase : simulink/Logic and Bit Operations/Compare To Constant  relop===  const=1  OutDataTypeStr=boolean
  Is weight shifted to the left side : RelationalOperator  Operator=>  OutDataTypeStr=boolean  RndMeth=Simplest
  Is weight shifted to the right side : RelationalOperator  Operator=<  OutDataTypeStr=boolean  RndMeth=Simplest
  Left leg is in flight : Logic  AllPortsSameDT=off  OutDataTypeStr=boolean
  Left leg torques : Selector  InputPortWidth=12  IndexOptions=Index vector (dialog)  Indices=[1:6]  OutputSizes=1
  Mux : Mux  Inputs=2
  Output left torques : Product
  Output right torques : Product
  Right leg is in flight : Logic  AllPortsSameDT=off  OutDataTypeStr=boolean
  Right leg torques : Selector  InputPortWidth=12  IndexOptions=Index vector (dialog)  Indices=[7:12]  OutputSizes=1
  Scope : Scope  NumInputPorts=4
  Switch : Switch  Criteria=u2 > Threshold
  Switch1 : Switch  Criteria=u2 > Threshold
  TL : Outport
  TR : Outport  Port=2
  wires:
  qL/1 -> Mux/1
  qR/1 -> Mux/2
  Mux/1 -> Gravity Torque/1
  phase_data/1 -> Bus Selector/1
  Gravity Torque/1 -> Left leg torques/1, Right leg torques/1
  Switch/1 -> TL/1
  Switch1/1 -> TR/1
  test_type/1 -> Inverse kinematics testing?/1
  Left leg torques/1 -> Output left torques/2, Switch/1
  Right leg torques/1 -> Output right torques/2, Switch1/1
  Inverse kinematics testing?/1 -> Scope/1, Switch1/2, Switch/2  "compensate_both"
  Bus Selector/2 -> Is it single support phase/1  "<phase>"
  Is it single support phase/1 -> Scope/2, Right leg is in flight/1, Left leg is in flight/1  "phase"
  Bus Selector/1 -> Demux/1  "<w>"
  Demux/2 -> Is weight shifted to the right side/2, Is weight shifted to the left side/2
  Demux/1 -> Is weight shifted to the right side/1, Is weight shifted to the left side/1
  Output left torques/1 -> Switch/3
  Is weight shifted to the right side/1 -> Left leg is in flight/2
  Is weight shifted to the left side/1 -> Right leg is in flight/2
  Output right torques/1 -> Switch1/3
  Left leg is in flight/1 -> Scope/3, Output left torques/1  "lleg"
  Right leg is in flight/1 -> Scope/4, Output right torques/1  "rleg"

== system bipedal_robot_CTRL2/Controller Version 2/Inverse kinematics optimization/Fmincon Ikine (Matlab) ==
  FSM : Inport  OutDataTypeStr=Bus: FSM_bus
  ctrl_cfg : Inport  Port=2  OutDataTypeStr=Bus: ctrl_cfg_rem_bus
  meas : Inport  Port=3  OutDataTypeStr=Bus: meas_bus
  cmds : Inport  Port=4  OutDataTypeStr=Bus: ikine_inp_bus
  jacobians : Inport  Port=5  OutDataTypeStr=Bus: jac_bus
  phase_data : Inport  Port=6  OutDataTypeStr=Bus: ph_data_bus
  cont_data : Inport  Port=7
  FmL : Inport  Port=8
  FmR : Inport  Port=9
  Feedack of integral of full solution : Delay  DelayLength=1  InitialCondition=ik_opt.q_ini  SampleTime=Ts
  Feedback of full solution : Delay  DelayLength=1  InitialCondition=ik_opt.qp_ini  SampleTime=Ts
  Full body IKine solver : MATLAB Function  TreatAsAtomicUnit=on
  Only select joint angles : Selector  InputPortWidth=18  IndexOptions=Index vector (dialog)  Indices=[7:18]  OutputSizes=1
  Only select joint angles (old) : Selector  InputPortWidth=18  IndexOptions=Index vector (dialog)  Indices=[7:18]  OutputSizes=1
  Only select joint velocities : Selector  InputPortWidth=18  IndexOptions=Index vector (dialog)  Indices=[7:18]  OutputSizes=1
  q_ref : Outport
  qp_ref : Outport  Port=2
  q_ref_old : Outport  Port=3
  wires:
  FSM/1 -> Full body IKine solver/1(FSM)
  Only select joint velocities/1 -> qp_ref/1
  Only select joint angles/1 -> q_ref/1
  Only select joint angles (old)/1 -> q_ref_old/1
  ctrl_cfg/1 -> Full body IKine solver/2(ctrl_cfg)
  Feedback of full solution/1 -> Full body IKine solver/9(qp_ini)
  Feedack of integral of full solution/1 -> Only select joint angles (old)/1, Full body IKine solver/8(q_ini)
  jacobians/1 -> Full body IKine solver/5(Jlist)
  phase_data/1 -> Full body IKine solver/6(phase)
  cmds/1 -> Full body IKine solver/4(cmds)
  meas/1 -> Full body IKine solver/3(meas)
  Full body IKine solver/1(q_ref) -> Only select joint angles/1, Feedack of integral of full solution/1
  Full body IKine solver/2(qp_ref) -> Only select joint velocities/1, Feedback of full solution/1
  cont_data/1 -> Full body IKine solver/7(cont_data)
  FmL/1 -> Full body IKine solver/10(FmL)
  FmR/1 -> Full body IKine solver/11(FmR)

== system bipedal_robot_CTRL2/Controller Version 2/Inverse kinematics optimization/OSQP Ikine (Matlab) ==
  FSM : Inport
  ctrl_cfg : Inport  Port=2
  meas : Inport  Port=3
  cmds : Inport  Port=4
  jacobians : Inport  Port=5
  phase_data : Inport  Port=6
  cont_data : Inport  Port=7
  FmL : Inport  Port=8
  FmR : Inport  Port=9
  q_ref : Outport
  qp_ref : Outport  Port=2
  q_ref_old : Outport  Port=3

== system bipedal_robot_CTRL2/Controller Version 2/Inverse kinematics optimization/qpOASES (C++) ==
  FSM : Inport
  ctrl_cfg : Inport  Port=2
  meas : Inport  Port=3
  cmds : Inport  Port=4
  jacobians : Inport  Port=5
  phase_data : Inport  Port=6
  cont_data : Inport  Port=7
  FmL : Inport  Port=8
  FmR : Inport  Port=9
  q_ref : Outport
  qp_ref : Outport  Port=2
  q_ref_old : Outport  Port=3

== system bipedal_robot_CTRL2/Controller Version 2/Trajectory Generation/(C++ impl) ==
  FSM : Inport
  zmp_curr : Inport  Port=2
  com_m : Inport  Port=3
  tg_data : Outport

== system bipedal_robot_CTRL2/Controller Version 2/Trajectory Generation/Preview Controller (simulink impl) ==
  FSM : Inport
  zmp_curr : Inport  Port=2
  com_m : Inport  Port=3
  Bus Creator : BusCreator  Inputs=6  OutDataTypeStr=Bus: tg_out_bus
  Constant : Constant  Value=0
  Constant1 : Constant  Value=tg.par.zc
  Demux : Demux  Outputs=2
  MATLAB Function : MATLAB Function  TreatAsAtomicUnit=on
  Mux{,1,3..5} (5 alike) : Mux  Inputs=3
  Mux2 : Mux  Inputs=2
  Preview controller X : biped_lib/Preview block  Pctrl=tg
  Preview controller Y : biped_lib/Preview block  Pctrl=tg
  Selector : Selector  InputPortWidth=9  IndexOptions=Index vector (dialog)  Indices=[1:3]  OutputSizes=1
  Selector1 : Selector  InputPortWidth=9  IndexOptions=Index vector (dialog)  Indices=[4:6]  OutputSizes=1
  X coord : Scope  NumInputPorts=4
  Y coord : Scope  NumInputPorts=4
  tg_data : Outport
  wires:
  Bus Creator/1 -> tg_data/1
  Constant1/1 -> Mux/3, Mux3/3
  Constant/1 -> Mux1/3, Mux5/3, Mux4/3
  Preview controller Y/4 -> Y coord/4, Mux5/2
  Preview controller X/4 -> Mux5/1, X coord/4
  Mux5/1 -> Bus Creator/4  "compp"
  Preview controller Y/3 -> Y coord/3, Mux4/2
  Preview controller X/3 -> Mux4/1, X coord/3
  Mux4/1 -> Bus Creator/3  "comp"
  Mux3/1 -> Bus Creator/2  "com"
  Preview controller Y/2 -> Y coord/2, Mux3/2
  Preview controller X/2 -> Mux3/1, X coord/2
  Mux1/1 -> Bus Creator/6  "dcmp"
  Mux/1 -> Bus Creator/5  "dcm"
  Mux2/1 -> Bus Creator/1  "zmp"
  Preview controller Y/1 -> Y coord/1, Mux2/2
  Preview controller X/1 -> Mux2/1, X coord/1
  Preview controller X/6 -> Mux1/1
  Preview controller X/5 -> Mux/1
  Preview controller Y/6 -> Mux1/2
  Preview controller Y/5 -> Mux/2
  MATLAB Function/2(use_meas) -> Preview controller X/4, Preview controller Y/4
  MATLAB Function/1(reset) -> Preview controller Y/2, Preview controller X/2
  FSM/1 -> MATLAB Function/1(FSM)
  Selector1/1 -> Preview controller Y/3
  Selector/1 -> Preview controller X/3
  com_m/1 -> Selector1/1, Selector/1
  Demux/2 -> Preview controller Y/1
  Demux/1 -> Preview controller X/1
  zmp_curr/1 -> Demux/1

== system bipedal_robot_CTRL2/Variant Subsystem/Floating base/Disturbance generator ==
  Constant : Constant  Value=0
  External Force and Torque : sm_lib/Forces and Torques/External Force and Torque  ForceResolutionFrame=World  EnableForceX=on  EnableForceY=on  EnableForceZ=on  EnableForce=off  TorqueResolutionFrame=World  EnableTorqueX=on  EnableTorqueY=on  EnableTorqueZ=on  EnableTorque=off
  Gain : Gain  Gain=VAR_DIST
  Simulink-PS Converter : nesl_utility/Simulink-PS Converter  PhysicalDomain=network_engine_domain  SubClassName=ps_input  LeftPortType=input  RightPortType=output  PseudoPeriodic=off  Frequencies=[]  NoiseDistribution=none  NoiseParameters=[]  Unit=1  AffineConversion=off  FilteringAndDerivatives=provide  SimscapeFilterOrder=2  InputFilterTimeConstant=0.001  UdotUserProvided=0
      settings: SourceProductName=Utilities
  Simulink-PS Converter1 : nesl_utility/Simulink-PS Converter  PhysicalDomain=network_engine_domain  SubClassName=ps_input  LeftPortType=input  RightPortType=output  PseudoPeriodic=off  Frequencies=[]  NoiseDistribution=none  NoiseParameters=[]  Unit=1  AffineConversion=off  FilteringAndDerivatives=zero  SimscapeFilterOrder=2  InputFilterTimeConstant=0.001  UdotUserProvided=0
      settings: SourceProductName=Utilities
  Step : Step  Time=Tdist(1)  After=Fdist(2)  SampleTime=0
  Step1 : Step  Time=Tdist(2)  After=Fdist(2)  SampleTime=0
  Sum : Sum  Inputs=|+-
  Disturbance : PMIOPort  Side=Right
  wires:
  Gain/1 -> Simulink-PS Converter1/1
  Constant/1 -> Simulink-PS Converter/1
  Step/1 -> Sum/1
  Step1/1 -> Sum/2
  Sum/1 -> Gain/1
  connections:
  Simulink-PS Converter1/RConn1 -- External Force and Torque/LConn2
  External Force and Torque/RConn1 -- Disturbance/RConn1
  Simulink-PS Converter/RConn1 -- External Force and Torque/LConn6 -- External Force and Torque/LConn5 -- External Force and Torque/LConn4 -- External Force and Torque/LConn3 -- External Force and Torque/LConn1

== matlab function bipedal_robot_CTRL2/Controller Version 2/Static spring force compensation (internal forces)/Gas spring compensation ==
  data: ctrl_cfg input; MSL input; MSR input; HL_list input; TL output; TR output; HR_list input
function [TL, TR] = fcn(ctrl_cfg, MSL, MSR, HL_list, HR_list)
    [LL,RL] = group_motor_data(MSL,MSR);
    qL = LL.q;
    qR = RL.q;
    consts = ctrl_cfg.sf_comp.gs;
    HL = HL_list;
    HR = HR_list;
    [TL, TR] = damperCompensTorques2(qL,qR,HL,HR,consts);
end

== matlab function bipedal_robot_CTRL2/Controller Version 2/State Estimation/FDkine ==
  data: ctrl_cfg input; Hw_b input; Jw_eeL output; Hb_L input; Hb_R input; Hb_comi input; Jw_eeR output; Jw_com output; Jw_b output; Jb_eeL output; Jb_eeR output
function [Jw_eeL, Jw_eeR, Jw_com, Jw_b, Jb_eeL, Jb_eeR]  = fcn(ctrl_cfg,Hw_b, Hb_L, Hb_R, Hb_comi)
    mlist = ctrl_cfg.fb_est.mlist;

    Nq = ctrl_cfg.par.Nq;
    Hb_i = zeros(Nq+2,4,4); 
    Hb_i(1:end/2,:,:) = Hb_L;
    Hb_i(end/2+1:end,:,:) = Hb_R;

    %% create jacobians
    % get com->base jacobians 
    Jb_comi = compute_com_jac_base(Nq,Hb_i,Hb_comi);

    % get ee->base jaccobian
    Jb_eeL = compute_jacobian(Hb_L,7);
    Jb_eeR = compute_jacobian(Hb_R,7);

    %% transform them to world jacobians and add a jacobian for the base
    frame_flag = 'b';
    % get com->world jacobians 
    Jw_comi = compute_jac_world2(Hw_b,Jb_comi,Hb_i,frame_flag);

    % get ee->world jacobian
    % left
    Hb_eeL = reshape(Hb_L(end,:,:),4,4);
    Jw_eeL_g = compute_jac_world_single2(Hw_b, Jb_eeL, Hb_eeL, 'l', frame_flag);
    % right
    Hb_eeR = reshape(Hb_R(end,:,:),4,4);
    Jw_eeR_g = compute_jac_world_single2(Hw_b, Jb_eeR, Hb_eeR, 'r', frame_flag);

    % get base->world jacobian
    Jw_b_g = compute_jac_world_single2(Hw_b, zeros(6,Nq/2), eye(4), 'b', frame_flag);
    
    %% compute com jacobian
    Jw_com_g = compute_centroidal_jac(Jw_comi,mlist);
    
    %% transform jacobians so that they are consistent with the configuration
    % account for the configuration dependent differences in mapping
    % between generalised and parametrised velocities
    eulconv = 'xyz';
    e = rotm2eul(Hw_b(1:3,1:3),eulconv);
    
    [Efx] = get_FB_matrix(e,Nq,eulconv);

    Jw_eeL_o = Jw_eeL_g * Efx;
    Jw_eeR_o = Jw_eeR_g * Efx;
    Jw_b_o   = Jw_b_g   * Efx;
    Jw_com_o = Jw_com_g * Efx;
    
    Jw_eeL = Jw_eeL_o(1:6,1:18);
    Jw_eeR = Jw_eeR_o(1:6,1:18);
    Jw_b = Jw_b_o(1:6,1:18);
    Jw_com = Jw_com_o(1:6,1:18);

end

== matlab function bipedal_robot_CTRL2/Controller Version 2/State Estimation/COM computation ==
  data: ctrl_cfg input; Hw_b input; Hb_comi input; zmp input; com output; comp output; compp output; dcm output; Jw_com input; dcmp output; Hb_c output
function [com, comp, compp, dcm, dcmp, Hb_c] = fcn(ctrl_cfg, Hw_b, Hb_comi, zmp, Jw_com)
persistent init com_old comp_old compp_old;

fb_est = ctrl_cfg.fb_est;
Ts = ctrl_cfg.par.Ts;
omega = fb_est.omega;
mlist = fb_est.mlist;

% IIR filter parameters
alpha_cp = fb_est.iir.alpha_cp;
alpha_cpp = fb_est.iir.alpha_cpp;

if isempty(init)
    init = 1;
    com_old = fb_est.init.com; %prevents controller jumps
    comp_old = zeros(3,1);
    compp_old = zeros(3,1);
end

% compute com position in base frame
com_b = compute_com_pos(Hb_comi,mlist);
Hb_c = [eye(3),com_b;zeros(1,3),1];

% get estimated com postion
com_w = Hw_b * [com_b;1];

% compute com outputs
com = com_w(1:3);
comp = alpha_cp*(com-com_old)/Ts + (1-alpha_cp)*comp_old;
compp = alpha_cpp*(comp-com_old)/Ts + (1-alpha_cpp)*compp_old;

% there is a possible way of computing the velocity using other data
% sources as well. Try it out if there is enough time.

% overwrite old values
com_old = com;
comp_old = comp;
compp_old = compp;

% compute dcm outputs
dcm = com + comp/omega;
dcmp = omega * (dcm - [zmp;0]);
dcmp_alt = comp + compp/omega; %alternative way of computing dcmp (lag version)

dcm_m = [dcm;dcmp];

== matlab function bipedal_robot_CTRL2/Controller Version 2/State Estimation/Global ZMP estimation ==
  data: Hw_b input; zmp output; FSL input; Hb_eeL input; FSR input; Hb_eeR input; zmpL output; zmpR output; ctrl_cfg input; cont_data output Bus: cd_bus
function [zmp,zmpL,zmpR,cont_data] = fcn(Hw_b, FSL,Hb_eeL, FSR, Hb_eeR, ctrl_cfg)
    Hw_eeL = Hw_b * Hb_eeL;
    Hw_eeR = Hw_b * Hb_eeR;
    
    % recompute ZMPs
    foot_data = ctrl_cfg.fb_est.foot_data;
    threshold_force = 1;
    simple_zmp = 0;
    [zmp,zmpL_full,zmpR_full,stateL,stateR] = compute_zmp_full2(FSL, FSR, foot_data, Hw_eeL, Hw_eeR, threshold_force, simple_zmp); %computed zmp
    if isnan(zmp)
        zmp = zeros(2,1);
    end
    zmpL = zmpL_full.glo;
    zmpR = zmpR_full.glo;
    
    [FL, FR, TL, TR, cL, cR] = compute_contact_data(FSL, FSR, stateL, stateR, ctrl_cfg);
    cont_data = create_cd_struct([zmpL_full.loc;0], [zmpR_full.loc;0], FL, FR, TL, TR, cL, cR, stateL, stateR);
    %cont_data = create_cd_struct(zeros(3,1), zeros(3,1), zeros(3,1), zeros(3,1), zeros(3,1), zeros(3,1), 0, 0);
end

== matlab function bipedal_robot_CTRL2/Controller Version 2/Static spring force compensation (internal forces)/Bungee cord compensation ==
  data: ctrl_cfg input; HL_list input; TL output; TR output; HR_list input
function [TL, TR] = fcn(ctrl_cfg, HL_list, HR_list)
    consts = ctrl_cfg.sf_comp.bc;
    HL = HL_list;
    HR = HR_list;
    [TL, TR] = bcordCompensTorques2(HL,HR,consts);
end

== matlab function bipedal_robot_CTRL2/Controller Version 2/Compute torques/Gain scheduling ==
  data: time input; FSM input; ctrl_cfg input; phase_data input; KpL output; KpR output; KdL output; KdR output; KiL output; KiR output; cont_data input; wGain input
function [KpL,KpR,KdL,KdR,KiL,KiR] = fcn(time, FSM, ctrl_cfg, phase_data, cont_data, wGain)
    % contact measurements
    contL = cont_data.L.cont;
    contR = cont_data.R.cont;

    test_type = ctrl_cfg.fsm.test_type;
    phase = phase_data.phase;
    w = phase_data.w;
    WshiftL = w(1);
    WshiftR = w(2);
    choice = 0;
    if choice==1
        [KpL, KpR, KdL, KdR] = get_gains3(FSM,test_type, phase, WshiftL, WshiftR, contL, contR);
    else
        [KpL, KpR, KdL, KdR] = get_gains4(test_type, wGain);
    end
    Ki = [100;100;100;100;20;20]*10;
    KiL = Ki;
    KiR = Ki;
    
    if time==0
        KpL = 0*KpL;
        KpR = 0*KpR;
        KdL = 0*KdL;
        KdR = 0*KdR;
    end
        
end
